simulink model "se_filter"  (Simulink 10.0)
settings: Solver=ode23tb  StartTime=0.0  StopTime=2.5  RelTol=1e-3  EnableMultiTasking=on
InitFcn:
  | Ts=20e-6;
undefined symbols (not defined in the file): DiscIntNeverNeededParam
libraries: powerlib x28, powerlib_extras x2
settings Model: Creator=srikanth  LastModifiedBy=bhisma
settings DataIOCC: LimitDataPoints=on  SignalLoggingSaveFormat=ModelDataLogs  SaveOutput=off  SaveTime=off
settings OptimizationCC: ExpressionDepthLimit=2147483647
settings DebuggingCC: AlgebraicLoopMsg=none  SolverPrmCheckMsg=warning  FcnCallInpInsideContextMsg=warning  StateNameClashWarn=warning
settings ConfigComp: CovExternalEMLEnable=off

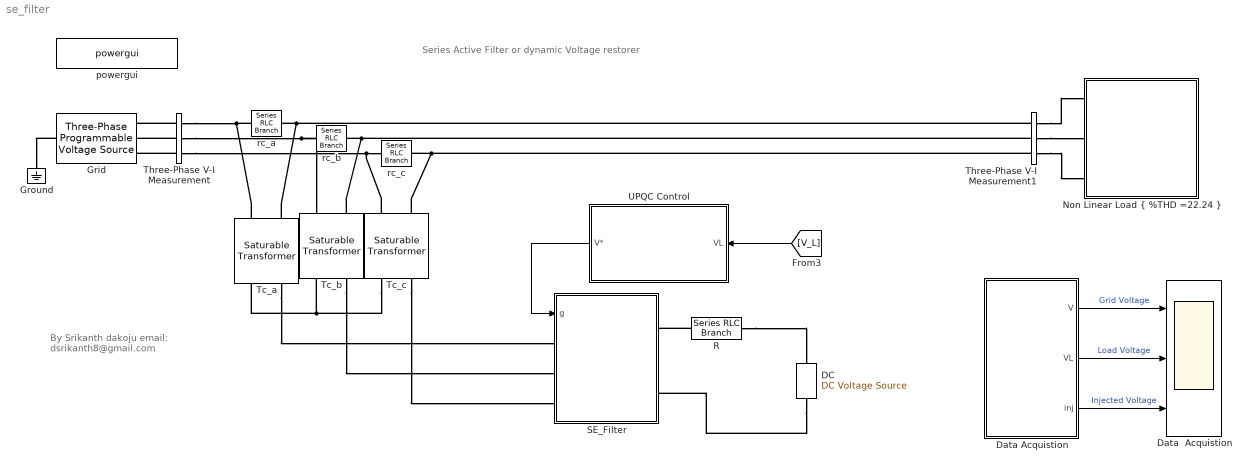
== system se_filter ==
  note: Series Active Filter or dynamic Voltage restorer
  note: By
      | Srikanth dakoju
      | email: dsrikanth8@gmail.com
  DC : powerlib/Electrical Sources/DC Voltage Source  SystemSampleTime=-1  Amplitude=700  Measurements=None
      settings: SourceProductName=Simscape Electrical
  Data  Acquistion : Scope  NumInputPorts=3
  Data Acquistion : Subsystem
      mask Display: fprintf('scopes')
  Grid : powerlib/Electrical Sources/Three-Phase Programmable Voltage Source  SystemSampleTime=-1  PositiveSequence="[380  0 50]"  VariationEntity=Amplitude  VariationType=Table of time-amplitude pairs  VariationStep=0.5  VariationRate=10  VariationMagnitude=0.3  VariationFrequency=2  VariationTiming=[1 2]  VariationPhaseA=off  Amplitudes=[1 0.5 1 1.5 1]  TimeValues=[0 0.5 0.7 1.5 1.7]  HarmonicGeneration=on  HarmonicA=[5 0.2 0 2]  HarmonicB=[7 0.05 0 1]  Timing="[0.2  0.4]"
      settings: SourceProductName=Simscape Electrical
  Ground : powerlib/Elements/Ground  PhysicalDomain=powersysdomain  SubClassName=unknown  LeftPortType=p1  RightPortType=p1  LConnTagsString=a
      settings: SourceProductName=Simscape Electrical
  "Non Linear Load { %THD =22.24 }" : Subsystem
      mask Display: fprintf('Non Linear\nLoad')
  R : powerlib/Elements/Series RLC Branch  PhysicalDomain=powersysdomain  SubClassName=unknown  LeftPortType=p1  RightPortType=p1  LConnTagsString=__new0  RConnTagsString=__new0  BranchType=R  Resistance=0.1  Inductance=1e-3  SetiL0=off  InitialCurrent=0  Capacitance=1e-6  Setx0=off  InitialVoltage=0  Measurements=None
      settings: SourceProductName=Simscape Electrical
  SE_Filter : Subsystem
      mask Display: fprintf('series\nfilter')
  Tc_a : powerlib/Elements/Saturable Transformer  SystemSampleTime=-1  ThreeWindings=off  UNITS=pu  NominalPower=[4000 50]  Winding1="[380  0.02  0.02 ]"  Winding2="[380  0.02  0.02]"  Winding3="[ 315e3  0.002  0.08 ]"  Saturation=[ 0 0 ;1.016 9.043]*1e-3  CoreLoss=[117 0]  Hysteresis=off  DataFile='hysteresis.mat'  Measurements=None  MoreParameters=off  BreakLoop=off  DataType=off  InitialFlux=0  TransfoNumber=1
      settings: SourceProductName=Simscape Electrical  SourceProductBaseCode=PS
  Tc_b : powerlib/Elements/Saturable Transformer  SystemSampleTime=-1  ThreeWindings=off  UNITS=pu  NominalPower=[4000 50]  Winding1="[380  0.02  0.02 ]"  Winding2="[380  0.02  0.02]"  Winding3="[ 315e3  0.002  0.08 ]"  Saturation=[ 0 0 ;1.016 9.043]*1e-3  CoreLoss=[117 0]  Hysteresis=off  DataFile='hysteresis.mat'  Measurements=None  MoreParameters=off  BreakLoop=off  DataType=off  InitialFlux=0  TransfoNumber=1
      settings: SourceProductName=Simscape Electrical  SourceProductBaseCode=PS
  Tc_c : powerlib/Elements/Saturable Transformer  SystemSampleTime=-1  ThreeWindings=off  UNITS=pu  NominalPower=[4000 50]  Winding1="[380  0.02  0.02 ]"  Winding2="[380  0.02  0.02]"  Winding3="[ 315e3  0.002  0.08 ]"  Saturation=[ 0 0 ;1.016 9.043]*1e-3  CoreLoss=[117 0]  Hysteresis=off  DataFile='hysteresis.mat'  Measurements=None  MoreParameters=off  BreakLoop=off  DataType=off  InitialFlux=0  TransfoNumber=1
      settings: SourceProductName=Simscape Electrical  SourceProductBaseCode=PS
  Three-Phase V-I Measurement : powerlib/Measurements/Three-Phase V-I Measurement  SystemSampleTime=-1  VoltageMeasurement=phase-to-ground  SetLabelV=on  LabelV=Vabc  Vpu=off  CurrentMeasurement=yes  SetLabelI=on  LabelI=Iabc  Ipu=off  Pbase=100e6  Vbase=500e3  OutputType=Complex  PhasorSimulation=off  PSBequivalent=0
      settings: SourceProductName=Simscape Electrical
  Three-Phase V-I Measurement1 : powerlib/Measurements/Three-Phase V-I Measurement  SystemSampleTime=-1  VoltageMeasurement=phase-to-ground  SetLabelV=on  LabelV=V_L  Vpu=off  CurrentMeasurement=yes  SetLabelI=on  LabelI=I_L  Ipu=off  Pbase=100e6  Vbase=500e3  OutputType=Complex  PhasorSimulation=off  PSBequivalent=0
      settings: SourceProductName=Simscape Electrical
  UPQC Control : Subsystem
      mask Display: fprintf('Series\nFilter')
  powergui : powerlib/powergui  Priority=1  SystemSampleTime=-1  SimulationMode=Discrete  SampleTime=Ts  frequency=60  SPID=off  DisableSnubberDevices=off  DisableRonSwitches=off  DisableVfSwitches=off  SwTol=0  Interpol=off  frequencyindice=50  echomessages=off  HookPort=off  DisplayEquations=off  FunctionMessages=off  EnableUseOfTLC=off  x0status=blocks  RestoreLinks=warning  Frange=[0:2:500]  Ylog=off  Xlog=on  ShowGrid=off  save=off  variable=ZData  structure=voltage_pi  ZoomFFT=off  StartTime=1.5  cycles=10  DisplayStyle=1  fundamental=50  FreqAxis=on  MaxFrequency=1000  frequencyindicesteady=1  RmsSteady=1  display=off  Ts=0  methode=off
      settings: SourceProductName=Simscape Electrical
  rc_a : powerlib/Elements/Series RLC Branch  PhysicalDomain=powersysdomain  SubClassName=unknown  LeftPortType=p1  RightPortType=p1  LConnTagsString=__new0  RConnTagsString=__new0  BranchType=RC  Resistance=1  Inductance=1e-3  SetiL0=off  InitialCurrent=0  Capacitance=100e-6  Setx0=off  InitialVoltage=0  Measurements=Branch voltage
      settings: SourceProductName=Simscape Electrical
  rc_b : powerlib/Elements/Series RLC Branch  PhysicalDomain=powersysdomain  SubClassName=unknown  LeftPortType=p1  RightPortType=p1  LConnTagsString=__new0  RConnTagsString=__new0  BranchType=RC  Resistance=1  Inductance=1e-3  SetiL0=off  InitialCurrent=0  Capacitance=100e-6  Setx0=off  InitialVoltage=0  Measurements=Branch voltage
      settings: SourceProductName=Simscape Electrical
  rc_c : powerlib/Elements/Series RLC Branch  PhysicalDomain=powersysdomain  SubClassName=unknown  LeftPortType=p1  RightPortType=p1  LConnTagsString=__new0  RConnTagsString=__new0  BranchType=RC  Resistance=1  Inductance=1e-3  SetiL0=off  InitialCurrent=0  Capacitance=100e-6  Setx0=off  InitialVoltage=0  Measurements=Branch voltage
      settings: SourceProductName=Simscape Electrical
  wires:
  [V_L] -> UPQC Control/1(VL)
  UPQC Control/1(V*) -> SE_Filter/1(g)
  Data Acquistion/1(V) -> Data  Acquistion/1  "Grid Voltage"
  Data Acquistion/2(VL) -> Data  Acquistion/2  "Load Voltage"
  Data Acquistion/3("inj ") -> Data  Acquistion/3  "Injected Voltage"
  connections:
  Three-Phase V-I Measurement1/LConn2 -- rc_b/LConn1 -- Tc_b/RConn2
  Three-Phase V-I Measurement1/LConn1 -- rc_a/LConn1 -- Tc_a/RConn2
  Grid/LConn1 -- Ground/LConn1
  Three-Phase V-I Measurement/LConn1 -- Grid/RConn1
  Three-Phase V-I Measurement/LConn2 -- Grid/RConn2
  Three-Phase V-I Measurement/LConn3 -- Grid/RConn3
  Three-Phase V-I Measurement1/RConn2 -- "Non Linear Load { %THD =22.24 }"/LConn2
  Three-Phase V-I Measurement1/LConn3 -- rc_c/LConn1 -- Tc_c/RConn2
  rc_a/RConn1 -- Three-Phase V-I Measurement/RConn1 -- Tc_a/RConn1
  rc_b/RConn1 -- Three-Phase V-I Measurement/RConn2 -- Tc_b/RConn1
  rc_c/RConn1 -- Three-Phase V-I Measurement/RConn3 -- Tc_c/RConn1
  Three-Phase V-I Measurement1/RConn3 -- "Non Linear Load { %THD =22.24 }"/LConn3
  Three-Phase V-I Measurement1/RConn1 -- "Non Linear Load { %THD =22.24 }"/LConn1
  Tc_a/LConn2 -- SE_Filter/LConn1
  Tc_b/LConn2 -- SE_Filter/LConn2
  Tc_c/LConn2 -- SE_Filter/LConn3
  Tc_c/LConn1 -- Tc_a/LConn1 -- Tc_b/LConn1
  R/LConn1 -- SE_Filter/RConn1
  R/RConn1 -- DC/RConn1
  DC/LConn1 -- SE_Filter/RConn2

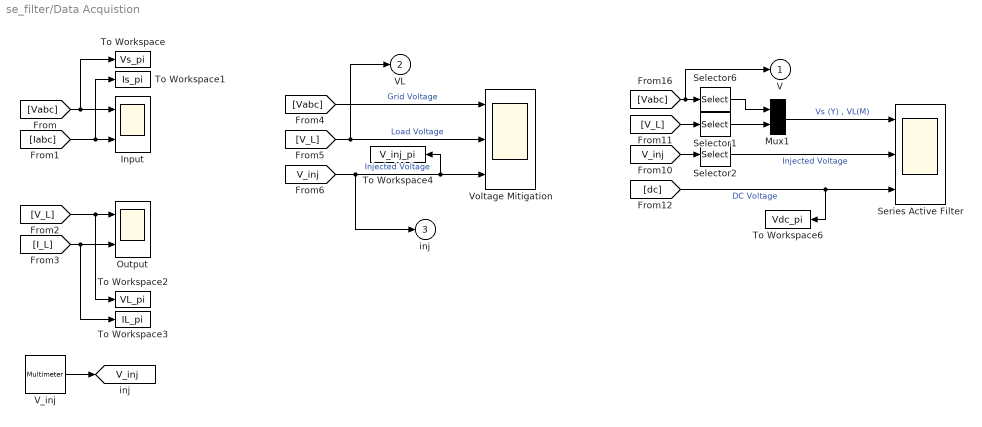
== system se_filter/Data Acquistion ==
  Input : Scope  NumInputPorts=2
  Mux1 : Mux  Inputs=2
      settings: DisplayOption=signals
  Output : Scope  NumInputPorts=2
  Selector1 : Selector  InputPortWidth=3  IndexOptions=Index vector (dialog)  Indices=1  OutputSizes=1
  Selector2 : Selector  InputPortWidth=3  IndexOptions=Index vector (dialog)  Indices=1  OutputSizes=1
  Selector6 : Selector  InputPortWidth=3  IndexOptions=Index vector (dialog)  Indices=1  OutputSizes=1
  Series Active Filter : Scope  NumInputPorts=3
  To Workspace : ToWorkspace  VariableName=Vs_pi  SampleTime=Ts
  To Workspace1 : ToWorkspace  VariableName=Is_pi  SampleTime=Ts
  To Workspace2 : ToWorkspace  VariableName=VL_pi  SampleTime=Ts
  To Workspace3 : ToWorkspace  VariableName=IL_pi  SampleTime=Ts
  To Workspace4 : ToWorkspace  VariableName=V_inj_pi  SampleTime=Ts
  To Workspace6 : ToWorkspace  VariableName=Vdc_pi  SampleTime=Ts
  V_inj : powerlib/Measurements/Multimeter  SystemSampleTime=-1  PhasorSimulation=off  OutputType=Complex  sel=[1 2 3]  L=3  Gain=[1 1 1]  yselected={'Ub: rc_a','Ub: rc_b','Ub: rc_c'};  PSBOutputType=1  PSBequivalent=0  AxesSetting=[0,0.1,-100,100]  Display=0  SavedBlockNames=-11
      settings: SourceProductName=Simscape Electrical
  Voltage Mitigation : Scope  NumInputPorts=3
  V : Outport
  VL : Outport  Port=2
  "inj " : Outport  Port=3
  tag scope: V_inj=global
  wires:
  [Vabc] -> Input/1, To Workspace/1
  [Iabc] -> Input/2, To Workspace1/1
  [V_L] -> Output/1, To Workspace2/1
  [I_L] -> Output/2, To Workspace3/1
  [Vabc] -> Voltage Mitigation/1  "Grid Voltage"
  [V_L] -> Voltage Mitigation/2, VL/1  "Load Voltage"
  [V_inj] -> Voltage Mitigation/3, To Workspace4/1, "inj "/1  "Injected Voltage"
  [V_L] -> Selector1/1
  [V_inj] -> Selector2/1
  [dc] -> Series Active Filter/3, To Workspace6/1  "DC Voltage"
  Selector2/1 -> Series Active Filter/2  "Injected Voltage"
  [Vabc] -> Selector6/1, V/1
  Selector1/1 -> Mux1/2
  Mux1/1 -> Series Active Filter/1  "Vs (Y) , VL(M)"
  Selector6/1 -> Mux1/1
  V_inj/1 -> [V_inj]

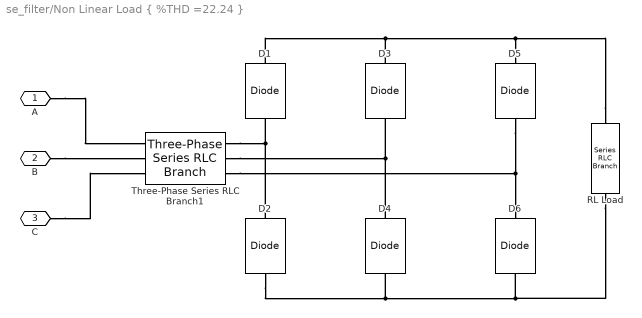
== system se_filter/Non Linear Load { %THD =22.24 } ==
  D{1..6} (6 alike) : powerlib/Power Electronics/Diode  SystemSampleTime=-1  Ron=0.001  Lon=0  Vf=0.8  IC=0  UseSnubber=off  Rs=500  Cs=250e-9  Measurements=off
      settings: SourceProductName=Simscape Electrical
  RL Load : powerlib/Elements/Series RLC Branch  PhysicalDomain=powersysdomain  SubClassName=unknown  LeftPortType=p1  RightPortType=p1  LConnTagsString=__new0  RConnTagsString=__new0  BranchType=RL  Resistance=60  Inductance=0.15e-3  SetiL0=off  InitialCurrent=0  Capacitance=1e-6  Setx0=off  InitialVoltage=0  Measurements=None
      settings: SourceProductName=Simscape Electrical
  Three-Phase Series RLC Branch1 : powerlib/Elements/Three-Phase Series RLC Branch  PhysicalDomain=powersysdomain  SubClassName=unknown  LeftPortType=p1  RightPortType=p1  LConnTagsString=A|B|C  RConnTagsString=A|B|C  BranchType=RL  Resistance=0.4  Inductance=15e-3  Capacitance=1e-6  Measurements=None
      settings: SourceProductName=Simscape Electrical
  A : PMIOPort  Side=Left
  B : PMIOPort  Port=2  Side=Left
  C : PMIOPort  Port=3  Side=Left
  connections:
  C/RConn1 -- Three-Phase Series RLC Branch1/LConn3
  B/RConn1 -- Three-Phase Series RLC Branch1/LConn2
  A/RConn1 -- Three-Phase Series RLC Branch1/LConn1
  Three-Phase Series RLC Branch1/RConn3 -- D6/RConn1 -- D5/LConn1
  Three-Phase Series RLC Branch1/RConn2 -- D4/RConn1 -- D3/LConn1
  RL Load/RConn1 -- D6/LConn1 -- D4/LConn1 -- D2/LConn1
  RL Load/LConn1 -- D5/RConn1 -- D3/RConn1 -- D1/RConn1
  Three-Phase Series RLC Branch1/RConn1 -- D2/RConn1 -- D1/LConn1

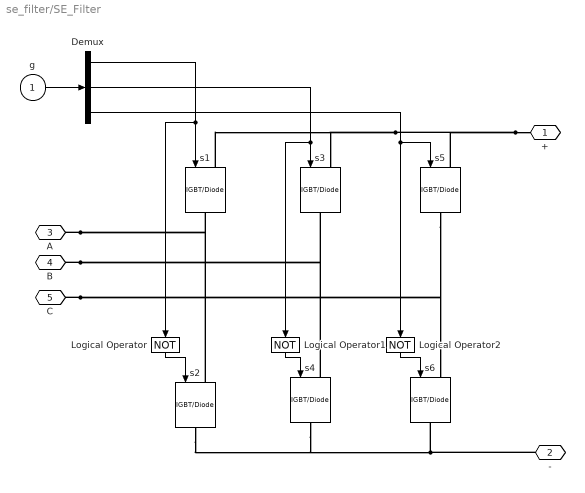
== system se_filter/SE_Filter ==
  g : Inport
  Demux : Demux  Outputs=3
  Logical Operator : Logic  Operator=NOT  AllPortsSameDT=off  OutDataTypeStr=boolean
  Logical Operator1 : Logic  Operator=NOT  AllPortsSameDT=off  OutDataTypeStr=boolean
  Logical Operator2 : Logic  Operator=NOT  AllPortsSameDT=off  OutDataTypeStr=boolean
  s{1..6} (6 alike) : powerlib/Power Electronics/IGBT//Diode  SystemSampleTime=-1  Ron=1e-3  Rs=1e5  Cs=inf  Measurements=off
      settings: SourceProductName=Simscape Electrical
  + : PMIOPort  Side=Right
  - : PMIOPort  Port=2  Side=Right
  A : PMIOPort  Port=3  Side=Left
  B : PMIOPort  Port=4  Side=Left
  C : PMIOPort  Port=5  Side=Left
  wires:
  Demux/2 -> s3/1, Logical Operator1/1
  Demux/1 -> s1/1, Logical Operator/1
  Logical Operator/1 -> s2/1
  Logical Operator1/1 -> s4/1
  Logical Operator2/1 -> s6/1
  Demux/3 -> Logical Operator2/1, s5/1
  g/1 -> Demux/1
  connections:
  +/RConn1 -- s5/LConn1 -- s1/LConn1 -- s3/LConn1
  A/RConn1 -- s2/LConn1 -- s1/RConn1
  -/RConn1 -- s6/RConn1 -- s4/RConn1 -- s2/RConn1
  B/RConn1 -- s4/LConn1 -- s3/RConn1
  C/RConn1 -- s5/RConn1 -- s6/LConn1

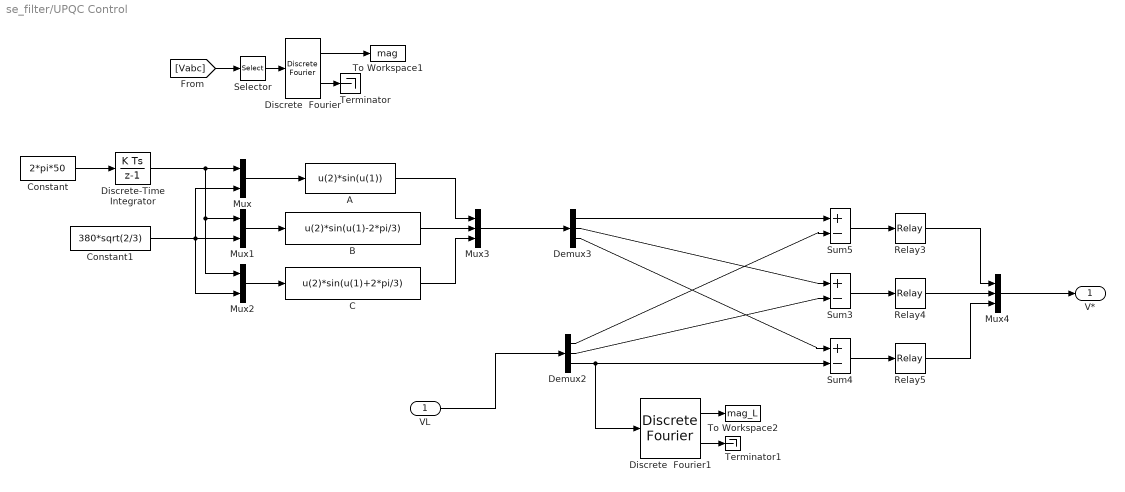
== system se_filter/UPQC Control ==
  VL : Inport
  A : Fcn  Expr=u(2)*sin(u(1))
  B : Fcn  Expr=u(2)*sin(u(1)-2*pi/3)
  C : Fcn  Expr=u(2)*sin(u(1)+2*pi/3)
  Constant : Constant  Value=2*pi*50
  Constant1 : Constant  Value=380*sqrt(2/3)
  Demux2 : Demux  Outputs=3
  Demux3 : Demux  Outputs=3
  Discrete  Fourier : powerlib_extras/Discrete Measurements/Discrete  Fourier  SystemSampleTime=-1  Freq=50  n=1  Par_Init=[0 0]  Ts=Ts
      settings: SourceProductName=Simscape Electrical  SourceProductBaseCode=PS
  Discrete  Fourier1 : powerlib_extras/Discrete Measurements/Discrete  Fourier  SystemSampleTime=-1  Freq=50  n=1  Par_Init=[0 0]  Ts=Ts
      settings: SourceProductName=Simscape Electrical  SourceProductBaseCode=PS
  Discrete-Time Integrator : DiscreteIntegrator  SampleTime=Ts  ICPrevOutput=DiscIntNeverNeededParam  ICPrevScaledInput=DiscIntNeverNeededParam
  Mux : Mux  Inputs=2
  Mux1 : Mux  Inputs=2
  Mux2 : Mux  Inputs=2
  Mux3 : Mux  Inputs=3
  Mux4 : Mux  Inputs=3
  Relay3 : Relay  OnSwitchValue=1  OffSwitchValue=-1
  Relay4 : Relay  OnSwitchValue=1  OffSwitchValue=-1
  Relay5 : Relay  OnSwitchValue=1  OffSwitchValue=-1
  Selector : Selector  InputPortWidth=3  IndexOptions=Index vector (dialog)  Indices=1  OutputSizes=1
  Sum3 : Sum  Inputs=+-
  Sum4 : Sum  Inputs=+-
  Sum5 : Sum  Inputs=+-
  Terminator : Terminator
  Terminator1 : Terminator
  To Workspace1 : ToWorkspace  VariableName=mag  SampleTime=Ts
  To Workspace2 : ToWorkspace  VariableName=mag_L  SampleTime=Ts
  V* : Outport
  wires:
  Constant/1 -> Discrete-Time Integrator/1
  Discrete-Time Integrator/1 -> Mux/1, Mux2/1, Mux1/1
  Constant1/1 -> Mux/2, Mux1/2, Mux2/2
  Mux/1 -> A/1
  Mux1/1 -> B/1
  Mux2/1 -> C/1
  Discrete  Fourier/2 -> Terminator/1
  Selector/1 -> Discrete  Fourier/1
  [Vabc] -> Selector/1
  Discrete  Fourier/1 -> To Workspace1/1
  A/1 -> Mux3/1
  B/1 -> Mux3/2
  C/1 -> Mux3/3
  Discrete  Fourier1/2 -> Terminator1/1
  Sum5/1 -> Relay3/1
  Sum3/1 -> Relay4/1
  Sum4/1 -> Relay5/1
  Relay3/1 -> Mux4/1
  Relay4/1 -> Mux4/2
  Relay5/1 -> Mux4/3
  Mux4/1 -> V*/1
  Discrete  Fourier1/1 -> To Workspace2/1
  VL/1 -> Demux2/1
  Demux3/1 -> Sum5/1
  Demux2/3 -> Sum4/2, Discrete  Fourier1/1
  Demux2/1 -> Sum5/2
  Demux3/3 -> Sum4/1
  Demux2/2 -> Sum3/2
  Demux3/2 -> Sum3/1
  Mux3/1 -> Demux3/1
